simulink subsystem "EcuacionesDiferenciales"  (R2023b)
settings: Solver=VariableStepAuto  StartTime=0.0  StopTime=10.0  RelTol=1e-3
undefined symbols (not defined in the file): B, J, K, L, R
settings Model: Creator=jaime  LastModifiedBy=jaime

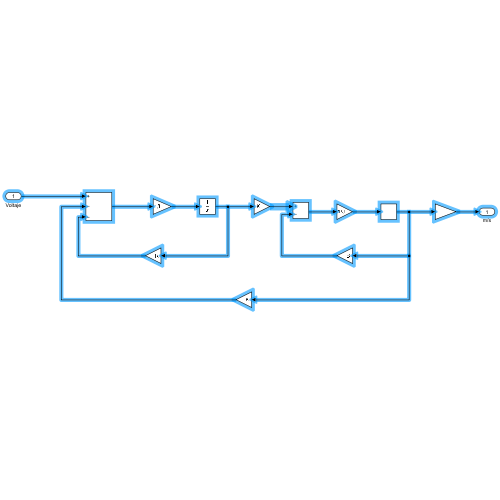
[thumbnail: Simulink's stored preview of the top-level diagram]
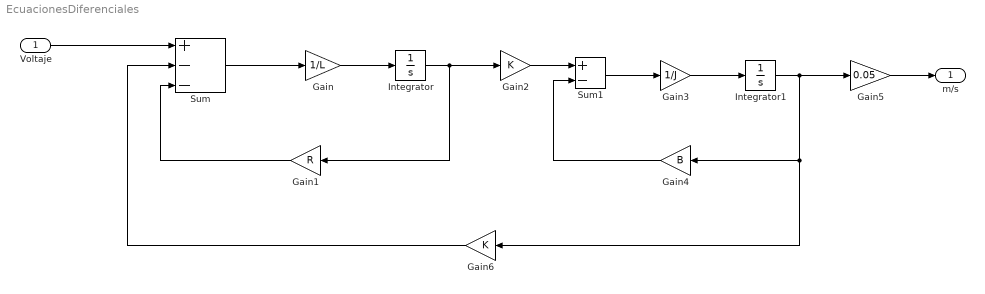
== system EcuacionesDiferenciales ==
  Voltaje : Inport
  Gain : Gain  Gain=1/L
  Gain1 : Gain  Gain=R
  Gain2 : Gain  Gain=K
  Gain3 : Gain  Gain=1/J
  Gain4 : Gain  Gain=B
  Gain5 : Gain  Gain=0.05
  Gain6 : Gain  Gain=K
  Integrator : Integrator
  Integrator1 : Integrator
  Sum : Sum  Inputs=+--
  Sum1 : Sum  Inputs=+-
  m/s : Outport
  wires:
  Sum1/1 -> Gain3/1
  Gain/1 -> Integrator/1
  Integrator/1 -> Gain1/1, Gain2/1
  Sum/1 -> Gain/1
  Voltaje/1 -> Sum/1
  Gain1/1 -> Sum/3
  Integrator1/1 -> Gain6/1, Gain4/1, Gain5/1
  Gain5/1 -> m/s/1
  Gain3/1 -> Integrator1/1
  Gain6/1 -> Sum/2
  Gain4/1 -> Sum1/2
  Gain2/1 -> Sum1/1
